simulink model "sl_subsys_trig1"  (Simulink 7.6)
settings: Solver=FixedStepDiscrete  SolverMode=SingleTasking  StartTime=0.0  StopTime=10.0  RelTol=1e-3
Description:
  | Latch vs. non-latched input ports example
settings Model: Creator=The MathWorks Inc.  CovMetricSettings=d  ExtModeAutoUpdateStatusClock=off
settings OptimizationCC: BlockReduction=off  BooleanDataType=off  InitFltsAndDblsToZero=on
settings DebuggingCC: SaveWithParameterizedLinksMsg=none  SignalResolutionControl=TryResolveAllWithWarning  SolverPrmCheckMsg=none  MultiTaskDSMMsg=warning  MultiTaskCondExecSysMsg=none
settings HardwareCC: TargetUnknown=on
settings RTWCC: IncludeERTFirstTime=on
settings CodeAppCC: CustomSymbolStrFcn=$F$N$M
settings GRTTargetCC: TargetFcnLib=ansi_tfl_tmw.mat

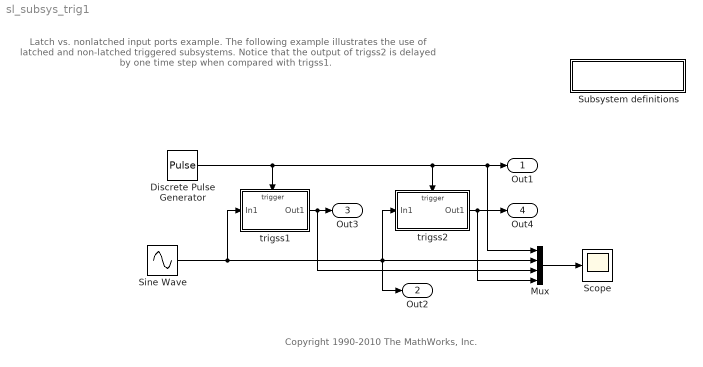
== system sl_subsys_trig1 ==
  note: Latch vs. nonlatched input ports example.
      |
      | The following example illustrates the use of latched
      | and non-latched triggered subsystems. Notice that
      | the output of trigss2 is delayed by one time step
      | when compared with trigss1.
  note: Copyright 1990-2010 The MathWorks, Inc.
  " Subsystem definitions" : Subsystem
      settings: OpenFcn=helpview([matlabroot,'/toolbox/simulink/simdemos/simfeatures/html/sl_subsys_definitions.html']);
      mask Display: disp('Subsystem\ndefinitions')
  Discrete Pulse Generator : DiscretePulseGenerator
  Mux : Mux
  Scope : Scope
  Sine Wave : Sin  SineType=Sample based  Amplitude=2  Samples=20  SampleTime=.25
  trigss1 : Subsystem  TreatAsAtomicUnit=on
  trigss2 : Subsystem  TreatAsAtomicUnit=on
  Out1 : Outport
  Out2 : Outport  Port=2
  Out3 : Outport  Port=3
  Out4 : Outport  Port=4
  wires:
  trigss1/1(Out1) -> Out3/1, Mux/3
  trigss2/1(Out1) -> Out4/1, Mux/4
  Discrete Pulse Generator/1 -> trigss1/Trigger, trigss2/Trigger, Out1/1, Mux/1
  Sine Wave/1 -> trigss1/1(In1), trigss2/1(In1), Out2/1, Mux/2
  Mux/1 -> Scope/1

== system sl_subsys_trig1/ Subsystem definitions ==

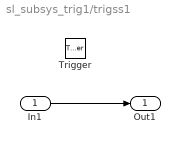
== system sl_subsys_trig1/trigss1 ==
  In1 : Inport
  Trigger : TriggerPort
  Out1 : Outport
  wires:
  In1/1 -> Out1/1

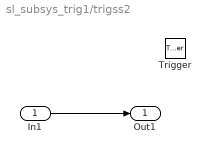
== system sl_subsys_trig1/trigss2 ==
  In1 : Inport  LatchByDelayingOutsideSignal=on
  Trigger : TriggerPort
  Out1 : Outport
  wires:
  In1/1 -> Out1/1
